simulink model "Tflex_PIDv1_ISSGP"  (R2018b)
settings: Solver=FixedStepDiscrete  StartTime=0.0  StopTime=inf  FixedStep=ts  RelTol=1e-3  EnableMultiTasking=on
PreLoadFcn:
  | Ts = 0.001;
InitFcn:
  | Ts = 0.001;
values from neighbouring files (symbols this model uses):
  a0 = omega_n^3    (= 31006276.6803)    [init_Tflex_PID_ISSGP.m]
  a1 = 3*omega_n^2    (= 296088.132033)    [init_Tflex_PID_ISSGP.m]
  a2 = 3*omega_n    (= 942.477796077)    [init_Tflex_PID_ISSGP.m]
  Avout = 10000    [init_Tflex_PID_ISSGP.m]
  b = ones(2*D,Q)*0.001    [init_Tflex_PID_ISSGP.m]
  D = 30    [init_Tflex_PID_ISSGP.m]
  FB1_offset = 1411500000    [init_Tflex_PID_ISSGP.m]
  h = 10*ts    (= 0.01)    [init_Tflex_PID_ISSGP.m]
  I_limit_max = 750    [init_Tflex_PID_ISSGP.m]
  I_limit_min = -250    [init_Tflex_PID_ISSGP.m]
  Kd = kp*(tau_z-tau_p*(1+(tau_z+tau_p)/tau_i))    [init_Tflex_PID_ISSGP.m]
  Ki = kp/tau_i    [init_Tflex_PID_ISSGP.m]
  Kp = kp*(1+(tau_z-tau_p)/tau_i)    [init_Tflex_PID_ISSGP.m]
  kp = m_eq*crossOver^2/sqrt(1/alpha)    [init_Tflex_PID_ISSGP.m]
  KTY_p0 = -146    [init_Tflex_PID_ISSGP.m]
  KTY_p1 = 263.3    [init_Tflex_PID_ISSGP.m]
  r = 1e2    (= 100)    [init_Tflex_PID_ISSGP.m]
  R = eye(2*D,2*D)*sn    [init_Tflex_PID_ISSGP.m]
  seed = 48125    [init_Tflex_PID_ISSGP.m]
  sf = 1.666976616732943e+05    (= 166697.661673)    [init_Tflex_PID_ISSGP.m]    (also in plot_Tflex_PIDv1_ISSGP18a.m = 500)
  sp_ts = 2    [init_Tflex_PID_ISSGP.m]
  tau_i = beta*tau_z    [init_Tflex_PID_ISSGP.m]
  tau_p = 1/(crossOver*sqrt(1/alpha))    [init_Tflex_PID_ISSGP.m]
  tau_z = sqrt(1/alpha)/crossOver    [init_Tflex_PID_ISSGP.m]
  tm = 1.5    [init_Tflex_PID_ISSGP.m]
  ts = 1/fs    (= 0.001)    [init_Tflex_PID_ISSGP.m]
  w = ones(2*D,Q)*0.001    [init_Tflex_PID_ISSGP.m]
undefined symbols (not defined in the file or in its folder): DiscIntNeverNeededParam, LPden, LPnum, SIGMA
libraries: xpcethercatlib x17, simulink x10, slrtlib x5
settings Model: SimulationMode=external  ExtModeTrigDirection=either  Creator=lab  LastModifiedBy=wout7
settings SolverCC: ConcurrentTasks=on  AutoInsertRateTranBlk=on
settings DataIOCC: LimitDataPoints=on  MaxDataPoints=50000  SaveFormat=StructureWithTime
settings OptimizationCC: BlockReduction=off  OptimizeBlockIOStorage=off  BufferReuse=off  GlobalBufferReuse=off  ExpressionFolding=off  LocalBlockOutputs=off  OptimizeDataStoreBuffers=off  BusAssignmentInplaceUpdate=off
settings DebuggingCC: UnconnectedInputMsg=none  UnconnectedOutputMsg=none  UnconnectedLineMsg=none  LibraryContextMissingDiagnostic=none
settings HardwareCC: ProdBitPerPointer=32  ProdBitPerSizeT=32  ProdBitPerPtrDiffT=32  ProdLargestAtomicFloat=None  ProdWordSize=32  ProdLongLongMode=on  ProdHWDeviceType=Generic->32-bit x86 compatible
settings SFSimCC: SimUserSources=dpotrs_wrapper.c;  SimUserLibraries=libmwlapack.lib  SimUseLocalCustomCode=off
settings SFSimCC: SimUserIncludeDirs=|
  | "C:\Program Files\MATLAB\R2018a\extern\lib\win64\microsoft"
  | "C:\Program Files\MATLAB\R2018a\bin\win64"
  | "C:\Users\wout7\Documents\GitHub\Inverse_dynamics_learning\TargetPC\Tflex PID 17-5-2019\TLC"
settings RTWCC: SystemTargetFile=slrt.tlc  TemplateMakefile=slrt_default_tmf  Description=Simulink Real-Time  RTWUseLocalCustomCode=off  CodeExecutionProfiling=on  RTWCompilerOptimization=on
settings SimulinkRealTimeCC: SupportVariableSizeSignals=on  PreserveStateflowLocalDataDimensions=off  xPCConcurrentTasks=on

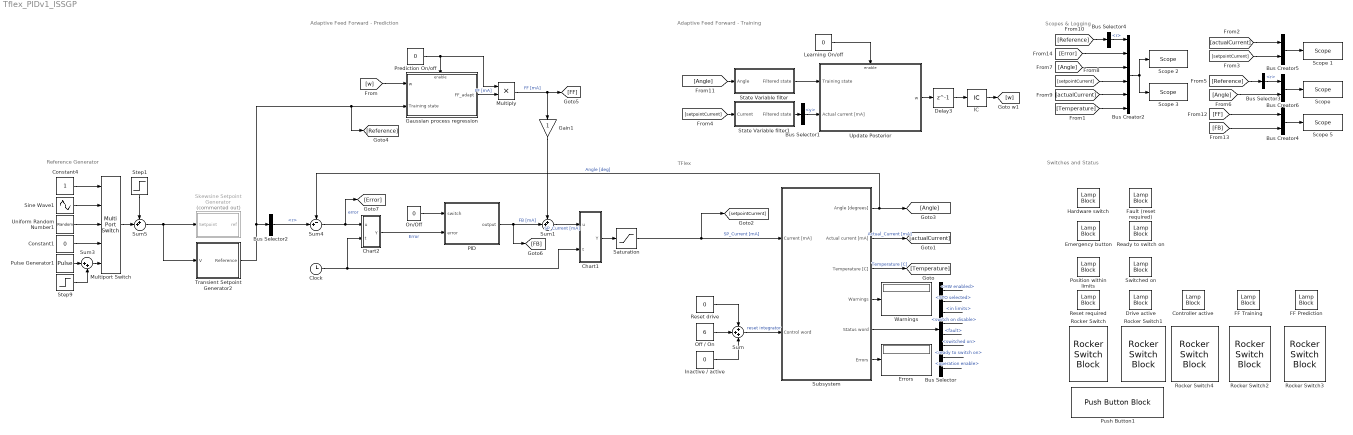
== system Tflex_PIDv1_ISSGP ==
  note: TFlex
  note: Switches and Status
  note: Scopes & Logging
  note: Adaptive Feed Forward - Prediction
  note: Reference Generator
  note: Adaptive Feed Forward - Training
  Bus Creator2 : BusCreator  Inputs=6
  Bus Creator4 : BusCreator  Inputs=2
  Bus Creator5 : BusCreator  Inputs=2
  Bus Creator6 : BusCreator  Inputs=2
  Bus Selector : BusSelector  OutputSignals=HW enabled,STO selected,in limits,switch on disable,fault,switched on,ready to switch on,operation enable
  Bus Selector1 : BusSelector  OutputSignals=y
  Bus Selector2 : BusSelector  OutputSignals=r
  Bus Selector3 : BusSelector  OutputSignals=r
  Bus Selector4 : BusSelector  OutputSignals=r
  Chart1 : Stateflow chart  TreatAsAtomicUnit=on
  Chart2 : Stateflow chart  TreatAsAtomicUnit=on
  Clock : Clock
  Constant1 : Constant  Value=0  SampleTime=sp_ts
  Constant4 : Constant  SampleTime=sp_ts
  Controller active : LampBlock  WebBlockId=1912  LabelPosition=Hide
  Delay3 : Delay  DelayLength=1  InitialCondition=0
  Drive active : LampBlock  WebBlockId=227
  Emergency button : LampBlock  WebBlockId=221
  Errors : Display
  FF Prediction : LampBlock  WebBlockId=1916  LabelPosition=Hide
  FF Training : LampBlock  WebBlockId=1915  LabelPosition=Hide
  Fault (reset required) : LampBlock  WebBlockId=224
  Gain1 : Gain
  Gaussian process regression : Subsystem
  Hardware switch : LampBlock  WebBlockId=218
  IC : InitialCondition  Value=w
  Inactive / active : Constant  Value=0
  Learning On/off : Constant  Value=0
  Multiply : Product
  Multiport Switch : MultiPortSwitch  Inputs=4
  Off / On : Constant  Value=6
  On/Off : Constant  Value=0
  "PID " : Subsystem
  Position within limits : LampBlock  WebBlockId=222
  Prediction On/off : Constant  Value=0  SampleTime=ts
  Pulse Generator1 : DiscretePulseGenerator  Amplitude=46  SampleTime=sp_ts
  Push Button1 : PushButtonBlock  WebBlockId=1977  ButtonText=Reset Drive [TURN OFF FIRST]  OnValue=128
  Ready to switch on : LampBlock  WebBlockId=226
  Reset drive : Constant  Value=0
  Reset required : LampBlock  WebBlockId=223
  Rocker Switch : RockerSwitchBlock  WebBlockId=231  LabelPosition=Hide
      settings: Values={{'Off', 'Driver On'}, [6 7]}
  Rocker Switch1 : RockerSwitchBlock  WebBlockId=232  LabelPosition=Hide
      settings: Values={{'Inactive', 'Driver Active'}, [0 8]}
  Rocker Switch2 : RockerSwitchBlock  WebBlockId=965  LabelPosition=Hide
      settings: Values={{'Off', 'Training on'}, [0 1]}
  Rocker Switch3 : RockerSwitchBlock  WebBlockId=969  LabelPosition=Hide
      settings: Values={{'Off', 'Prediction On'}, [0 1]}
  Rocker Switch4 : RockerSwitchBlock  WebBlockId=1848  LabelPosition=Hide
      settings: Values={{'Off', 'Controller On'}, [0 1]}
  Saturation : Saturate  UpperLimit=750  LowerLimit=-250/2
  "Scope " : slrtlib/Displays and Logging/Scope   scopeno=1  scopetype=Target  autostart=on  viewmode=Graphical redraw  formatstr='%15.6f'  grid=on  ylimits=[0 ,0]  nosamples=2000  noprepostsamples=0  interleave=1  triggermode=FreeRun  triggersignal=1  trigsignalfromport=off  triggerlevel=0.0  triggerslope=Either  triggerscope=1  triggersample=0  filename=data.dat  mode=Lazy  writesize=512  autorestart=off  dynamicfilemode=off  maxwritefilesize=512*1024^2
  Scope 1 : slrtlib/Displays and Logging/Scope   scopeno=2  scopetype=Target  autostart=on  viewmode=Graphical redraw  formatstr='%15.6f'  grid=on  ylimits=[500,500]  nosamples=250  noprepostsamples=0  interleave=1  triggermode=FreeRun  triggersignal=1  trigsignalfromport=off  triggerlevel=0.0  triggerslope=Either  triggerscope=1  triggersample=0  filename=data.dat  mode=Lazy  writesize=512  autorestart=off  dynamicfilemode=off  maxwritefilesize=512*1024^2
  Scope 2 : slrtlib/Displays and Logging/Scope   scopeno=3  scopetype=Target  autostart=on  viewmode=Numerical  formatstr='%15.6f,%15.6f,%15.6f,%15.0f'  grid=on  ylimits=[500,500]  nosamples=250  noprepostsamples=0  interleave=1  triggermode=FreeRun  triggersignal=1  trigsignalfromport=off  triggerlevel=0.0  triggerslope=Either  triggerscope=1  triggersample=0  filename=data.dat  mode=Lazy  writesize=512  autorestart=off  dynamicfilemode=off  maxwritefilesize=512*1024^2
  Scope 3 : slrtlib/Displays and Logging/Scope   scopeno=6  scopetype=File  autostart=on  viewmode=Graphical redraw  formatstr='%15.6f'  grid=on  ylimits=[0,0]  nosamples=600000  noprepostsamples=0  interleave=1  triggermode=FreeRun  triggersignal=1  trigsignalfromport=off  triggerlevel=0.0  triggerslope=Either  triggerscope=1  triggersample=0  filename=data.dat  mode=Lazy  writesize=512  autorestart=off  dynamicfilemode=off  maxwritefilesize=512*1024^2
  Scope 5 : slrtlib/Displays and Logging/Scope   scopeno=5  scopetype=Target  autostart=on  viewmode=Graphical redraw  formatstr='%15.6f'  grid=on  ylimits=[500,500]  nosamples=250  noprepostsamples=0  interleave=1  triggermode=FreeRun  triggersignal=1  trigsignalfromport=off  triggerlevel=0.0  triggerslope=Either  triggerscope=1  triggersample=0  filename=data.dat  mode=Lazy  writesize=512  autorestart=off  dynamicfilemode=off  maxwritefilesize=512*1024^2
  Sine Wave1 : Sin  Amplitude=15  Frequency=2*pi*2  SampleTime=0
  Skewsine Setpoint Generator : Subsystem  Commented=on
  State Variable filter : Subsystem
  State Variable filter1 : Subsystem
  Step1 : Step  Time=20  Before=-23  After=0  SampleTime=0
  Step9 : Step  Time=0  After=-24  SampleTime=sp_ts
  Subsystem : Subsystem
  Sum : Sum  Inputs=+++
  Sum1 : Sum  Inputs=++|
  Sum3 : Sum  Inputs=|++
  Sum4 : Sum  Inputs=-+|
  Sum5 : Sum  Inputs=++|
  Switched on : LampBlock  WebBlockId=225
  Transient Setpoint Generator2 : Subsystem
  Uniform Random Number1 : UniformRandomNumber  Seed=seed  SampleTime=sp_ts
  Update Posterior : Subsystem
  Warnings : Display
  wires:
  Subsystem/2(Actual current [mA]) -> [actualCurrent]  "Actual_Current [mA]"
  Subsystem/5(Status word) -> Bus Selector/1
  Bus Selector/1 -> ?  "<HW enabled>"
  Bus Selector/2 -> ?  "<STO selected>"
  Bus Selector/3 -> ?  "<in limits>"
  Bus Selector/4 -> ?  "<switch on disable>"
  Bus Selector/5 -> ?  "<fault>"
  Bus Selector/6 -> ?  "<switched on>"
  Bus Selector/7 -> ?  "<ready to switch on>"
  Bus Selector/8 -> ?  "<operation enable>"
  Reset drive/1 -> Sum/1
  Off / On/1 -> Sum/2
  Inactive / active/1 -> Sum/3
  Subsystem/3(Temperature [C]) -> [Temperature]  "Temperature [C]"
  Subsystem/4(Warnings) -> Warnings/1
  Subsystem/6(Errors) -> Errors/1
  Sum/1 -> Subsystem/2(Control word)  "reset integrator"
  Subsystem/1(Angle [degrees]) -> [Angle], Sum4/1  "Angle [deg]"
  Chart1/1(Y) -> Saturation/1
  Sum1/1 -> Chart1/1(u)  "SP_Current [mA]"
  Chart2/1(Y) -> "PID "/2(error)  "Error"
  Sum4/1 -> [Error], Chart2/1(u)  "error"
  Clock/1 -> Chart2/2(t), Chart1/2(t)
  State Variable filter/1(Filtered state) -> Update Posterior/1(Training state)
  IC/1 -> [w]
  Delay3/1 -> IC/1
  Update Posterior/1(w) -> Delay3/1
  [w] -> Gaussian process regression/1(w)
  Prediction On/off/1 -> Gaussian process regression/Enable, Multiply/1
  Learning On/off/1 -> Update Posterior/Enable
  Bus Creator4/1 -> Scope 5/1
  Uniform Random Number1/1 -> Multiport Switch/3
  Sine Wave1/1 -> Multiport Switch/2
  Constant4/1 -> Multiport Switch/1
  Transient Setpoint Generator2/1(Reference) -> Gaussian process regression/2(Training state), [Reference], Bus Selector2/1
  Sum5/1 -> Skewsine Setpoint Generator/1(Setpoint), Transient Setpoint Generator2/1(V)
  Gain1/1 -> Sum1/1
  Multiply/1 -> Gain1/1, [FF]  "FF [mA]"
  Gaussian process regression/1(FF_adapt) -> Multiply/2  "FF [mA]"
  State Variable filter1/1(Filtered state) -> Bus Selector1/1
  Bus Selector1/1 -> Update Posterior/2("Actual current [mA] ")  "<y>"
  [setpointCurrent] -> State Variable filter1/1(Current)
  [actualCurrent] -> Bus Creator5/1
  [setpointCurrent] -> Bus Creator5/2
  Bus Creator5/1 -> Scope 1/1
  [Reference] -> Bus Selector3/1
  [Angle] -> Bus Creator6/2
  Bus Selector3/1 -> Bus Creator6/1  "<r>"
  Bus Creator6/1 -> "Scope "/1
  [Reference] -> Bus Selector4/1
  [Angle] -> Bus Creator2/3
  [setpointCurrent] -> Bus Creator2/4
  [actualCurrent] -> Bus Creator2/5
  [Temperature] -> Bus Creator2/6
  Bus Creator2/1 -> Scope 2/1, Scope 3/1
  [Angle] -> State Variable filter/1(Angle)
  "PID "/1(output) -> [FB], Sum1/2  "FB [mA]"
  [FF] -> Bus Creator4/1
  [FB] -> Bus Creator4/2
  Bus Selector2/1 -> Sum4/2  "<r>"
  [Error] -> Bus Creator2/2
  Saturation/1 -> [setpointCurrent], Subsystem/1(Current [mA])  "SP_Current [mA]"
  Bus Selector4/1 -> Bus Creator2/1  "<r>"
  On/Off/1 -> "PID "/1(switch)
  Multiport Switch/1 -> Sum5/2
  Step1/1 -> Sum5/1
  Pulse Generator1/1 -> Sum3/1
  Step9/1 -> Sum3/2
  Sum3/1 -> Multiport Switch/5
  Constant1/1 -> Multiport Switch/4

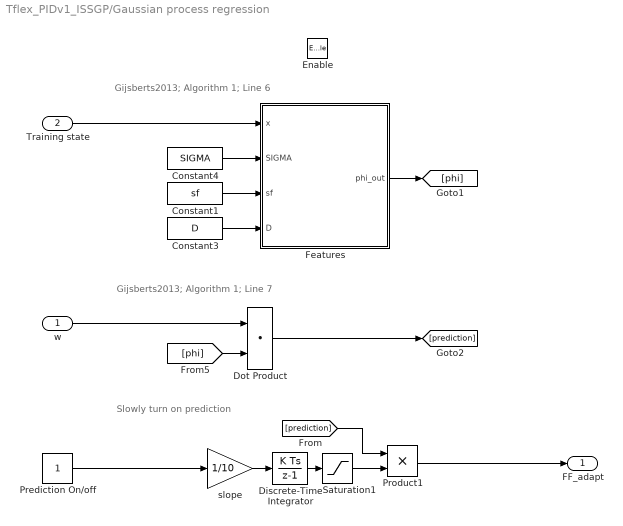
== system Tflex_PIDv1_ISSGP/Gaussian process regression ==
  note: Gijsberts2013; Algorithm 1; Line 7
  note: Gijsberts2013; Algorithm 1; Line 6
  note: Slowly turn on prediction
  w : Inport
  Training state : Inport  Port=2
  Enable : EnablePort  StatesWhenEnabling=reset
  Constant1 : Constant  Value=sf  VectorParams1D=off
  Constant3 : Constant  Value=D  VectorParams1D=off
  Constant4 : Constant  Value=SIGMA  VectorParams1D=off
  Discrete-Time Integrator : DiscreteIntegrator  SampleTime=-1  ICPrevOutput=DiscIntNeverNeededParam  ICPrevScaledInput=DiscIntNeverNeededParam
  Dot Product : DotProduct  OutDataTypeStr=Inherit: Inherit via internal rule
  Features : Subsystem
  Prediction On/off : Constant
  Product1 : Product
  Saturation1 : Saturate  UpperLimit=1  LowerLimit=0
  slope : Gain  Gain=1/10
  FF_adapt : Outport  SampleTime=ts
  wires:
  w/1 -> Dot Product/1
  [phi] -> Dot Product/2
  Product1/1 -> FF_adapt/1
  slope/1 -> Discrete-Time Integrator/1
  Prediction On/off/1 -> slope/1
  Discrete-Time Integrator/1 -> Saturation1/1
  Dot Product/1 -> [prediction]
  Constant4/1 -> Features/2(SIGMA)
  Training state/1 -> Features/1(x)
  Features/1(phi_out) -> [phi]
  Constant3/1 -> Features/4(D)
  Constant1/1 -> Features/3(sf)
  Saturation1/1 -> Product1/2
  [prediction] -> Product1/1

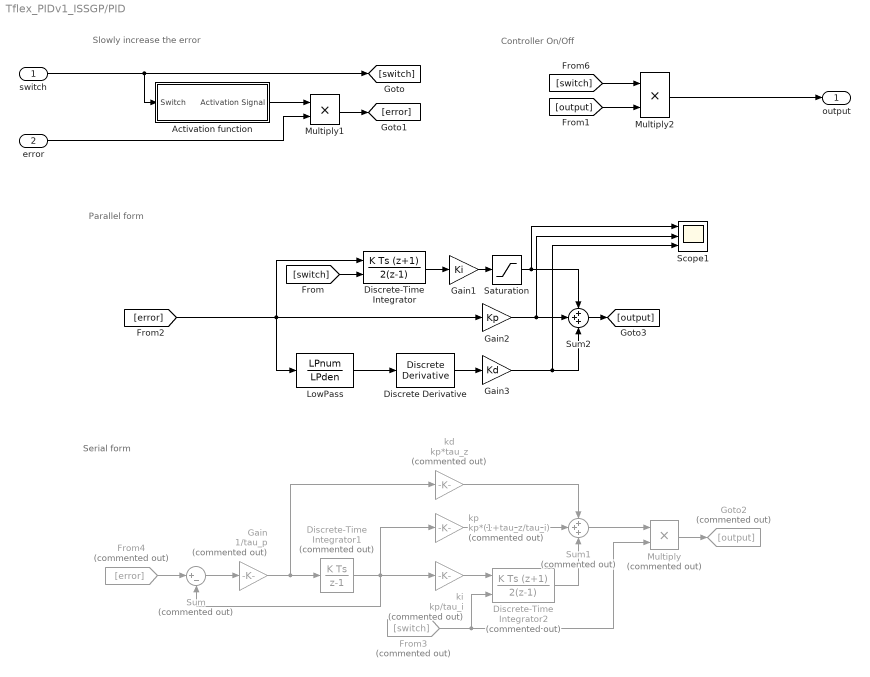
== system Tflex_PIDv1_ISSGP/PID  ==
  note: Controller On/Off
  note: Slowly increase the error
  note: Serial form
  note: Parallel form
  switch : Inport  SampleTime=ts
  error : Inport  Port=2
  Activation function : Subsystem
  Discrete Derivative : simulink/Discrete/Discrete Derivative  gainval=1.0  ICPrevScaledInput=0.0  OutMin=[]  OutMax=[]  OutDataType=fixdt(1, 16)  OutScaling=2^-10  DoSatur=off
  Discrete-Time Integrator : DiscreteIntegrator  IntegratorMethod=Integration: Trapezoidal  ExternalReset=either  SampleTime=ts  LimitOutput=on  UpperSaturationLimit=I_limit_max  LowerSaturationLimit=I_limit_min  ICPrevOutput=DiscIntNeverNeededParam  ICPrevScaledInput=DiscIntNeverNeededParam
  Discrete-Time Integrator1 : DiscreteIntegrator  Commented=on  SampleTime=-1  ICPrevOutput=DiscIntNeverNeededParam  ICPrevScaledInput=DiscIntNeverNeededParam
  Discrete-Time Integrator2 : DiscreteIntegrator  Commented=on  IntegratorMethod=Integration: Trapezoidal  ExternalReset=rising  SampleTime=ts  LimitOutput=on  UpperSaturationLimit=I_limit_max  LowerSaturationLimit=I_limit_min  ICPrevOutput=DiscIntNeverNeededParam  ICPrevScaledInput=DiscIntNeverNeededParam
  From3 : From  Commented=on  GotoTag=switch
  From4 : From  Commented=on  GotoTag=error
  Gain : Gain  Commented=on  Gain=1/tau_p
  Gain1 : Gain  Gain=Ki
  Gain2 : Gain  Gain=Kp
  Gain3 : Gain  Gain=Kd
  Goto2 : Goto  Commented=on  GotoTag=output
  LowPass : DiscreteTransferFcn  Numerator=LPnum  Denominator=LPden
  Multiply : Product  Commented=on
  Multiply1 : Product
  Multiply2 : Product
  Saturation : Saturate  UpperLimit=I_limit_max  LowerLimit=I_limit_min
  Scope1 : Scope  NumInputPorts=3
  Sum : Sum  Commented=on  Inputs=|+-
  Sum1 : Sum  Commented=on  Inputs=+++
  Sum2 : Sum  Inputs=+++
  kd : Gain  Commented=on  Gain=kp*tau_z
  ki : Gain  Commented=on  Gain=kp/tau_i
  kp : Gain  Commented=on  Gain=kp*(1+tau_z/tau_i)
  output : Outport
  wires:
  LowPass/1 -> Discrete Derivative/1
  [error] -> Discrete-Time Integrator/1, Gain2/1, LowPass/1
  Discrete-Time Integrator/1 -> Gain1/1
  Gain2/1 -> Scope1/2, Sum2/2
  Gain3/1 -> Scope1/3, Sum2/3
  Sum2/1 -> [output]
  Sum/1 -> Gain/1
  Gain/1 -> Discrete-Time Integrator1/1, kd/1
  ki/1 -> Discrete-Time Integrator2/1
  Discrete-Time Integrator1/1 -> kp/1, ki/1, Sum/2
  kp/1 -> Sum1/2
  kd/1 -> Sum1/1
  Discrete-Time Integrator2/1 -> Sum1/3
  Discrete Derivative/1 -> Gain3/1
  From4/1 -> Sum/1
  Sum1/1 -> Multiply/1
  From3/1 -> Discrete-Time Integrator2/2, Multiply/2
  Multiply/1 -> Goto2/1
  switch/1 -> [switch], Activation function/1(Switch)
  error/1 -> Multiply1/2
  [output] -> Multiply2/2
  [switch] -> Discrete-Time Integrator/2
  Multiply1/1 -> [error]
  [switch] -> Multiply2/1
  Multiply2/1 -> output/1
  Saturation/1 -> Sum2/1, Scope1/1
  Gain1/1 -> Saturation/1
  Activation function/1(Activation Signal) -> Multiply1/1

== system Tflex_PIDv1_ISSGP/Skewsine Setpoint Generator ==
  Setpoint : Inport
  Bus Creator : BusCreator  Inputs=3
  Delay : Delay  Commented=through  DelayLength=1  InitialCondition=0
  Subsystem : Subsystem
  ref : Outport
  wires:
  Subsystem/3(r_ddot) -> Bus Creator/3  "r_ddot"
  Bus Creator/1 -> ref/1
  Setpoint/1 -> Delay/1
  Subsystem/2(r_dot) -> Bus Creator/2  "r_dot"
  Subsystem/1(r) -> Bus Creator/1  "r"
  Delay/1 -> Subsystem/1(setpoint)

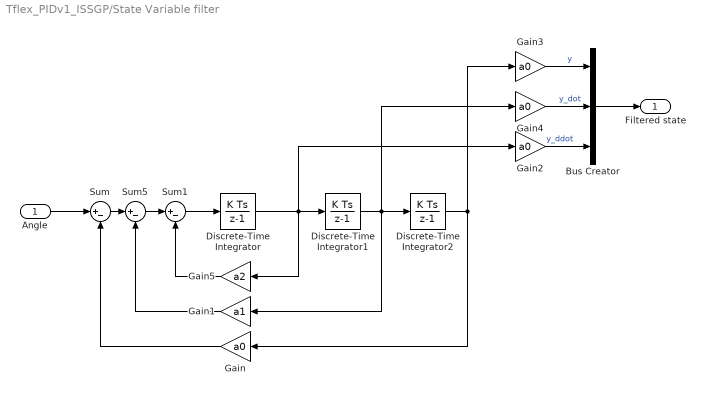
== system Tflex_PIDv1_ISSGP/State Variable filter ==
  Angle : Inport
  Bus Creator : BusCreator  Inputs=3
  Discrete-Time Integrator : DiscreteIntegrator  SampleTime=-1  ICPrevOutput=DiscIntNeverNeededParam  ICPrevScaledInput=DiscIntNeverNeededParam
  Discrete-Time Integrator1 : DiscreteIntegrator  SampleTime=-1  ICPrevOutput=DiscIntNeverNeededParam  ICPrevScaledInput=DiscIntNeverNeededParam
  Discrete-Time Integrator2 : DiscreteIntegrator  SampleTime=-1  ICPrevOutput=DiscIntNeverNeededParam  ICPrevScaledInput=DiscIntNeverNeededParam
  Gain{,2..4} (4 alike) : Gain  Gain=a0
  Gain1 : Gain  Gain=a1
  Gain5 : Gain  Gain=a2
  Sum : Sum  Inputs=|+-
  Sum1 : Sum  Inputs=|+-
  Sum5 : Sum  Inputs=|+-
  Filtered state : Outport
  wires:
  Bus Creator/1 -> Filtered state/1
  Angle/1 -> Sum/1
  Sum/1 -> Sum5/1
  Gain/1 -> Sum/2
  Gain1/1 -> Sum5/2
  Gain3/1 -> Bus Creator/1  "y"
  Gain2/1 -> Bus Creator/3  "y_ddot"
  Gain4/1 -> Bus Creator/2  "y_dot"
  Gain5/1 -> Sum1/2
  Sum5/1 -> Sum1/1
  Sum1/1 -> Discrete-Time Integrator/1
  Discrete-Time Integrator/1 -> Discrete-Time Integrator1/1, Gain2/1, Gain5/1
  Discrete-Time Integrator1/1 -> Discrete-Time Integrator2/1, Gain4/1, Gain1/1
  Discrete-Time Integrator2/1 -> Gain3/1, Gain/1

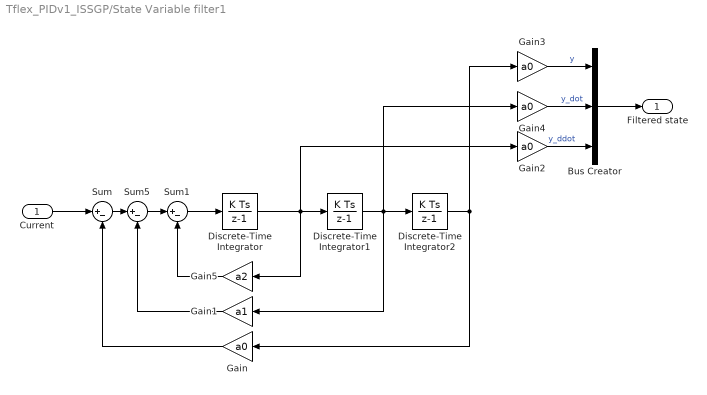
== system Tflex_PIDv1_ISSGP/State Variable filter1 ==
  Current : Inport
  Bus Creator : BusCreator  Inputs=3
  Discrete-Time Integrator : DiscreteIntegrator  SampleTime=-1  ICPrevOutput=DiscIntNeverNeededParam  ICPrevScaledInput=DiscIntNeverNeededParam
  Discrete-Time Integrator1 : DiscreteIntegrator  SampleTime=-1  ICPrevOutput=DiscIntNeverNeededParam  ICPrevScaledInput=DiscIntNeverNeededParam
  Discrete-Time Integrator2 : DiscreteIntegrator  SampleTime=-1  ICPrevOutput=DiscIntNeverNeededParam  ICPrevScaledInput=DiscIntNeverNeededParam
  Gain{,2..4} (4 alike) : Gain  Gain=a0
  Gain1 : Gain  Gain=a1
  Gain5 : Gain  Gain=a2
  Sum : Sum  Inputs=|+-
  Sum1 : Sum  Inputs=|+-
  Sum5 : Sum  Inputs=|+-
  Filtered state : Outport
  wires:
  Bus Creator/1 -> Filtered state/1
  Current/1 -> Sum/1
  Sum/1 -> Sum5/1
  Gain/1 -> Sum/2
  Gain1/1 -> Sum5/2
  Gain3/1 -> Bus Creator/1  "y"
  Gain2/1 -> Bus Creator/3  "y_ddot"
  Gain4/1 -> Bus Creator/2  "y_dot"
  Gain5/1 -> Sum1/2
  Sum5/1 -> Sum1/1
  Sum1/1 -> Discrete-Time Integrator/1
  Discrete-Time Integrator/1 -> Discrete-Time Integrator1/1, Gain2/1, Gain5/1
  Discrete-Time Integrator1/1 -> Discrete-Time Integrator2/1, Gain4/1, Gain1/1
  Discrete-Time Integrator2/1 -> Gain3/1, Gain/1

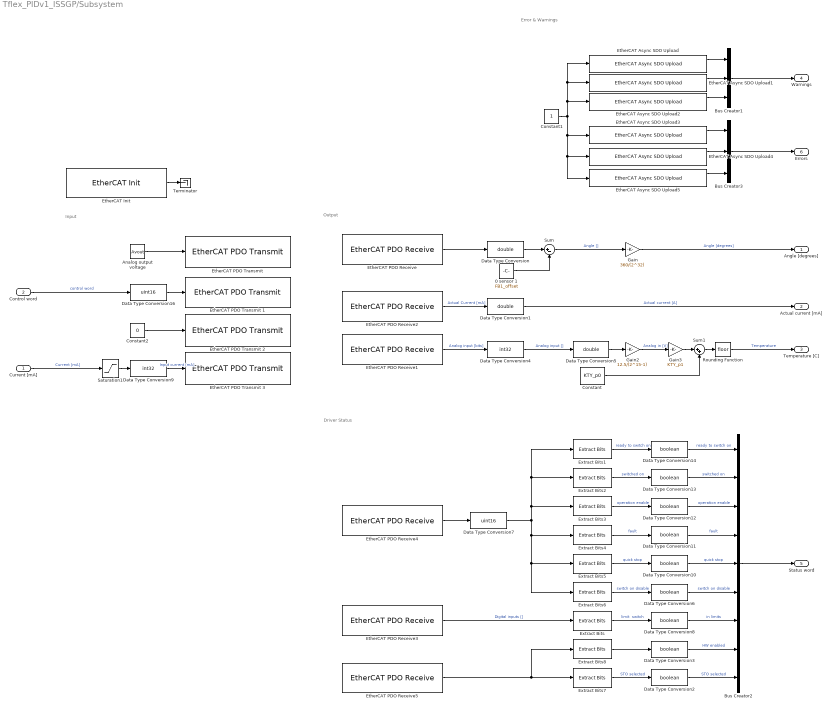
== system Tflex_PIDv1_ISSGP/Subsystem ==
  note: Output
  note: Error & Warnings
  note: Driver Status
  note: Input
  Current [mA] : Inport
  Control word : Inport  Port=2
  0 sensor 1 : Constant  Value=FB1_offset
  Analog output voltage : Constant  Value=Avout  OutDataTypeStr=int16
  Bus Creator1 : BusCreator  Inputs=3
  Bus Creator2 : BusCreator  Inputs=9
  Bus Creator3 : BusCreator  Inputs=3
  Constant : Constant  Value=KTY_p0
  Constant1 : Constant  OutDataTypeStr=int32
  Constant2 : Constant  Value=0  OutDataTypeStr=uint32
  Data Type Conversion : DataTypeConversion  OutDataTypeStr=double
  Data Type Conversion1 : DataTypeConversion  OutDataTypeStr=double
  Data Type Conversion{2..3,6,8,10..14} (9 alike) : DataTypeConversion  OutDataTypeStr=boolean
  Data Type Conversion16 : DataTypeConversion  OutDataTypeStr=uint16
  Data Type Conversion4 : DataTypeConversion  OutDataTypeStr=int32
  Data Type Conversion5 : DataTypeConversion  OutDataTypeStr=double
  Data Type Conversion7 : DataTypeConversion  OutDataTypeStr=uint16  RndMeth=Round
  Data Type Conversion9 : DataTypeConversion  OutDataTypeStr=int32
  EtherCAT Async SDO Upload : xpcethercatlib/EtherCAT Async SDO Upload  index=8192  subIndex=1  sig_type=uint32  sig_dim=1  device_id=0  slave_name=Drive 1 (AKD)  sample_time=1  slave_addr=1001  selected_slave=Term 1 (EK1100)  timeout=500  slave_found=1
      settings: SourceProductName=Simulink Real-Time  SourceProductBaseCode=XP
  EtherCAT Async SDO Upload1 : xpcethercatlib/EtherCAT Async SDO Upload  index=8192  subIndex=2  sig_type=uint32  sig_dim=1  device_id=0  slave_name=Drive 1 (AKD)  sample_time=1  slave_addr=1001  selected_slave=Term 1 (EK1100)  timeout=500  slave_found=1
      settings: SourceProductName=Simulink Real-Time  SourceProductBaseCode=XP
  EtherCAT Async SDO Upload2 : xpcethercatlib/EtherCAT Async SDO Upload  index=8192  subIndex=3  sig_type=uint32  sig_dim=1  device_id=0  slave_name=Drive 1 (AKD)  sample_time=1  slave_addr=1001  selected_slave=Term 1 (EK1100)  timeout=500  slave_found=1
      settings: SourceProductName=Simulink Real-Time  SourceProductBaseCode=XP
  EtherCAT Async SDO Upload3 : xpcethercatlib/EtherCAT Async SDO Upload  index=8193  subIndex=1  sig_type=uint32  sig_dim=1  device_id=0  slave_name=Drive 1 (AKD)  sample_time=1  slave_addr=1001  selected_slave=Term 1 (EK1100)  timeout=500  slave_found=1
      settings: SourceProductName=Simulink Real-Time  SourceProductBaseCode=XP
  EtherCAT Async SDO Upload4 : xpcethercatlib/EtherCAT Async SDO Upload  index=8193  subIndex=2  sig_type=uint32  sig_dim=1  device_id=0  slave_name=Drive 1 (AKD)  sample_time=1  slave_addr=1001  selected_slave=Term 1 (EK1100)  timeout=500  slave_found=1
      settings: SourceProductName=Simulink Real-Time  SourceProductBaseCode=XP
  EtherCAT Async SDO Upload5 : xpcethercatlib/EtherCAT Async SDO Upload  index=8193  subIndex=3  sig_type=uint32  sig_dim=1  device_id=0  slave_name=Drive 1 (AKD)  sample_time=1  slave_addr=1001  selected_slave=Term 1 (EK1100)  timeout=500  slave_found=1
      settings: SourceProductName=Simulink Real-Time  SourceProductBaseCode=XP
  "EtherCAT Init " : xpcethercatlib/EtherCAT Init   Priority=0  config_file=C:\Users\wout7\Documents\GitHub\Inverse_dynamics_learning\TargetPC\Tflex PID 17-5-2019\custom_pdo_eni3.xml  device_id=0  pci_bus=13  pci_slot=0  pci_function=0  initstate=2  dctuning=0  enaDebug=off  enaDC=on  errLink=off  masterDbg=off  stateChgDbg=off  baseClock=off  masterCfg=off  logFile='c:\dbglog.txt'  sample_time=0.001000  DCMode=2
      settings: SourceProductName=Simulink Real-Time  SourceProductBaseCode=XP
  EtherCAT PDO Receive : xpcethercatlib/EtherCAT PDO Receive  Priority=2  sig_name=Drive 1 (AKD).TPDO mapping parameter 3.Position actual internal value  sig_offset=624  sig_type=int32  type_size=32  sig_dim=1  device_id=0  sample_time=0.001000
      settings: SourceProductName=Simulink Real-Time  SourceProductBaseCode=XP
  EtherCAT PDO Receive1 : xpcethercatlib/EtherCAT PDO Receive  Priority=2  sig_name=Drive 1 (AKD).TPDO mapping parameter 1.AOUT_INPUT_VALUE  sig_offset=480  sig_type=int16  type_size=16  sig_dim=1  device_id=0  sample_time=0.001
      settings: SourceProductName=Simulink Real-Time  SourceProductBaseCode=XP
  EtherCAT PDO Receive2 : xpcethercatlib/EtherCAT PDO Receive  Priority=2  sig_name=Drive 1 (AKD).TPDO mapping parameter 2.Current actual value  sig_offset=528  sig_type=int32  type_size=32  sig_dim=1  device_id=0  sample_time=0.001000
      settings: SourceProductName=Simulink Real-Time  SourceProductBaseCode=XP
  EtherCAT PDO Receive3 : xpcethercatlib/EtherCAT PDO Receive  Priority=2  sig_name=Drive 1 (AKD).TPDO mapping parameter 1.Digital inputs  sig_offset=496  sig_type=uint32  type_size=32  sig_dim=1  device_id=0  sample_time=0.001000
      settings: SourceProductName=Simulink Real-Time  SourceProductBaseCode=XP
  EtherCAT PDO Receive4 : xpcethercatlib/EtherCAT PDO Receive  Priority=2  sig_name=Drive 1 (AKD).TPDO mapping parameter 1.Statusword  sig_offset=464  sig_type=uint16  type_size=16  sig_dim=1  device_id=0  sample_time=0.001
      settings: SourceProductName=Simulink Real-Time  SourceProductBaseCode=XP
  EtherCAT PDO Receive5 : xpcethercatlib/EtherCAT PDO Receive  Priority=2  sig_name=Drive 1 (AKD).TPDO mapping parameter 3.Manufacturer status register  sig_offset=592  sig_type=uint32  type_size=32  sig_dim=1  device_id=0  sample_time=0.001000
      settings: SourceProductName=Simulink Real-Time  SourceProductBaseCode=XP
  "EtherCAT PDO Transmit " : xpcethercatlib/EtherCAT PDO Transmit   Priority=3  sig_name=Drive 1 (AKD).RPDO mapping parameter 1.AOUT.VALUE write  sig_offset=480  sig_type=int16  type_size=16  sig_dim=1  device_id=0  sample_time=0.001000
      settings: SourceProductName=Simulink Real-Time  SourceProductBaseCode=XP
  EtherCAT PDO Transmit 1 : xpcethercatlib/EtherCAT PDO Transmit   Priority=3  sig_name=Drive 1 (AKD).RPDO mapping parameter 1.Controlword  sig_offset=464  sig_type=uint16  type_size=16  sig_dim=1  device_id=0  sample_time=0.001000
      settings: SourceProductName=Simulink Real-Time  SourceProductBaseCode=XP
  EtherCAT PDO Transmit 2 : xpcethercatlib/EtherCAT PDO Transmit   Priority=3  sig_name=Drive 1 (AKD).RPDO mapping parameter 1.Physical outputs  sig_offset=496  sig_type=uint32  type_size=32  sig_dim=1  device_id=0  sample_time=0.001000
      settings: SourceProductName=Simulink Real-Time  SourceProductBaseCode=XP
  EtherCAT PDO Transmit 3 : xpcethercatlib/EtherCAT PDO Transmit   Priority=3  sig_name=Drive 1 (AKD).RPDO mapping parameter 2.Target current  sig_offset=528  sig_type=int32  type_size=32  sig_dim=1  device_id=0  sample_time=0.001000
      settings: SourceProductName=Simulink Real-Time  SourceProductBaseCode=XP
  Extract Bits : simulink/Logic and Bit Operations/Extract Bits  bitsToExtract=Range of bits  numBits=8  bitIdxRange=[16]  outScalingMode=Treat bit field as an integer
      settings: SourceProductName=Simulink
  Extract Bits1 : simulink/Logic and Bit Operations/Extract Bits  bitsToExtract=Range of bits  numBits=8  bitIdxRange=[0]  outScalingMode=Treat bit field as an integer
      settings: SourceProductName=Simulink
  Extract Bits2 : simulink/Logic and Bit Operations/Extract Bits  bitsToExtract=Range of bits  numBits=8  bitIdxRange=[1]  outScalingMode=Treat bit field as an integer
      settings: SourceProductName=Simulink
  Extract Bits3 : simulink/Logic and Bit Operations/Extract Bits  bitsToExtract=Range of bits  numBits=8  bitIdxRange=[2]  outScalingMode=Treat bit field as an integer
      settings: SourceProductName=Simulink
  Extract Bits4 : simulink/Logic and Bit Operations/Extract Bits  bitsToExtract=Range of bits  numBits=8  bitIdxRange=[3]  outScalingMode=Treat bit field as an integer
      settings: SourceProductName=Simulink
  Extract Bits5 : simulink/Logic and Bit Operations/Extract Bits  bitsToExtract=Range of bits  numBits=8  bitIdxRange=[5]  outScalingMode=Treat bit field as an integer
      settings: SourceProductName=Simulink
  Extract Bits6 : simulink/Logic and Bit Operations/Extract Bits  bitsToExtract=Range of bits  numBits=8  bitIdxRange=[6]  outScalingMode=Treat bit field as an integer
      settings: SourceProductName=Simulink
  Extract Bits7 : simulink/Logic and Bit Operations/Extract Bits  bitsToExtract=Range of bits  numBits=8  bitIdxRange=[13]  outScalingMode=Treat bit field as an integer
      settings: SourceProductName=Simulink
  Extract Bits8 : simulink/Logic and Bit Operations/Extract Bits  bitsToExtract=Range of bits  numBits=8  bitIdxRange=[29]  outScalingMode=Treat bit field as an integer
      settings: SourceProductName=Simulink
  Gain : Gain  Gain=360/(2^32)
  Gain2 : Gain  Gain=12.5/(2^15-1)
  Gain3 : Gain  Gain=KTY_p1
  Rounding Function : Rounding
  Saturation1 : Saturate  UpperLimit=I_limit_max  LowerLimit=I_limit_min
  Sum : Sum  Inputs=|+-
  Sum1 : Sum  Inputs=|++  OutDataTypeStr=double
  Terminator : Terminator
  Angle [degrees] : Outport
  Actual current [mA] : Outport  Port=2
  Temperature [C] : Outport  Port=3
  Warnings : Outport  Port=4
  Status word : Outport  Port=5
  Errors : Outport  Port=6
  wires:
  Data Type Conversion/1 -> Sum/1
  Data Type Conversion9/1 -> EtherCAT PDO Transmit 3/1  "Input current [mA]"
  Bus Creator2/1 -> Status word/1
  0 sensor 1/1 -> Sum/2
  Data Type Conversion1/1 -> Actual current [mA]/1  "Actual current [A]"
  Data Type Conversion7/1 -> Extract Bits4/1, Extract Bits5/1, Extract Bits6/1, Extract Bits1/1, Extract Bits2/1, Extract Bits3/1
  EtherCAT PDO Receive4/1 -> Data Type Conversion7/1
  EtherCAT PDO Receive2/1 -> Data Type Conversion1/1  "Actual Current [mA]"
  Data Type Conversion4/1 -> Data Type Conversion5/1  "Analog input []"
  EtherCAT PDO Receive/1 -> Data Type Conversion/1
  Gain/1 -> Angle [degrees]/1  "Angle [degrees]"
  EtherCAT PDO Receive5/1 -> Extract Bits8/1, Extract Bits7/1
  EtherCAT PDO Receive1/1 -> Data Type Conversion4/1  "Analog input [bits]"
  Sum/1 -> Gain/1  "Angle []"
  Extract Bits8/1 -> Data Type Conversion3/1
  Extract Bits6/1 -> Data Type Conversion6/1  "switch on disable"
  Extract Bits/1 -> Data Type Conversion8/1  "limit  switch"
  Extract Bits3/1 -> Data Type Conversion12/1  "operation enable"
  Extract Bits2/1 -> Data Type Conversion13/1  "switched on"
  Extract Bits4/1 -> Data Type Conversion11/1  "fault"
  Extract Bits5/1 -> Data Type Conversion10/1  "quick stop"
  Constant2/1 -> EtherCAT PDO Transmit 2/1
  Extract Bits1/1 -> Data Type Conversion14/1  "ready to switch on"
  EtherCAT PDO Receive3/1 -> Extract Bits/1  "Digital inputs []"
  Extract Bits7/1 -> Data Type Conversion2/1  "STO selected"
  Data Type Conversion16/1 -> EtherCAT PDO Transmit 1/1
  "EtherCAT Init "/1 -> Terminator/1
  Data Type Conversion5/1 -> Gain2/1
  Analog output voltage/1 -> "EtherCAT PDO Transmit "/1
  Gain2/1 -> Gain3/1  "Analog in [V]"
  Sum1/1 -> Rounding Function/1
  Rounding Function/1 -> Temperature [C]/1  "Temperature"
  EtherCAT Async SDO Upload/1 -> Bus Creator1/1
  Bus Creator1/1 -> Warnings/1
  Constant1/1 -> EtherCAT Async SDO Upload5/1, EtherCAT Async SDO Upload4/1, EtherCAT Async SDO Upload3/1, EtherCAT Async SDO Upload/1, EtherCAT Async SDO Upload1/1, EtherCAT Async SDO Upload2/1
  EtherCAT Async SDO Upload1/1 -> Bus Creator1/2
  EtherCAT Async SDO Upload2/1 -> Bus Creator1/3
  EtherCAT Async SDO Upload3/1 -> Bus Creator3/1
  EtherCAT Async SDO Upload4/1 -> Bus Creator3/2
  EtherCAT Async SDO Upload5/1 -> Bus Creator3/3
  Bus Creator3/1 -> Errors/1
  Saturation1/1 -> Data Type Conversion9/1
  Gain3/1 -> Sum1/1
  Constant/1 -> Sum1/2
  Data Type Conversion8/1 -> Bus Creator2/7  "in limits"
  Data Type Conversion3/1 -> Bus Creator2/8  "HW enabled"
  Data Type Conversion10/1 -> Bus Creator2/5  "quick stop"
  Data Type Conversion6/1 -> Bus Creator2/6  "switch on disable"
  Data Type Conversion11/1 -> Bus Creator2/4  "fault"
  Data Type Conversion12/1 -> Bus Creator2/3  "operation enable"
  Data Type Conversion13/1 -> Bus Creator2/2  "switched on"
  Data Type Conversion2/1 -> Bus Creator2/9  "STO selected"
  Data Type Conversion14/1 -> Bus Creator2/1  "ready to switch on"
  Control word/1 -> Data Type Conversion16/1  "control word"
  Current [mA]/1 -> Saturation1/1  "Current [mA]"

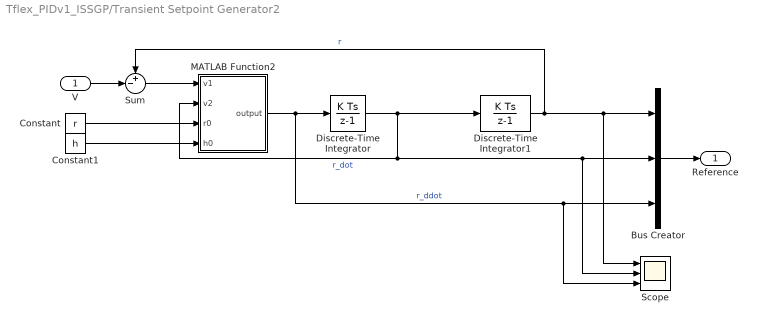
== system Tflex_PIDv1_ISSGP/Transient Setpoint Generator2 ==
  V : Inport
  Bus Creator : BusCreator  Inputs=3
  Constant : Constant  Value=r  SampleTime=ts
  Constant1 : Constant  Value=h  SampleTime=ts
  Discrete-Time Integrator : DiscreteIntegrator  gainval=1  SampleTime=ts  ICPrevOutput=DiscIntNeverNeededParam  ICPrevScaledInput=DiscIntNeverNeededParam
  Discrete-Time Integrator1 : DiscreteIntegrator  gainval=1  SampleTime=ts  ICPrevOutput=DiscIntNeverNeededParam  ICPrevScaledInput=DiscIntNeverNeededParam
  MATLAB Function2 : MATLAB Function  TreatAsAtomicUnit=on
  Scope : Scope  NumInputPorts=3
  Sum : Sum  Inputs=+-|
  Reference : Outport
  wires:
  Sum/1 -> MATLAB Function2/1(v1)
  V/1 -> Sum/2
  Constant/1 -> MATLAB Function2/3(r0)
  Constant1/1 -> MATLAB Function2/4(h0)
  Discrete-Time Integrator1/1 -> Scope/1, Bus Creator/1, Sum/1  "r"
  Discrete-Time Integrator/1 -> Discrete-Time Integrator1/1, MATLAB Function2/2(v2), Scope/2, Bus Creator/2  "r_dot"
  Bus Creator/1 -> Reference/1
  MATLAB Function2/1(output) -> Scope/3, Bus Creator/3, Discrete-Time Integrator/1  "r_ddot"

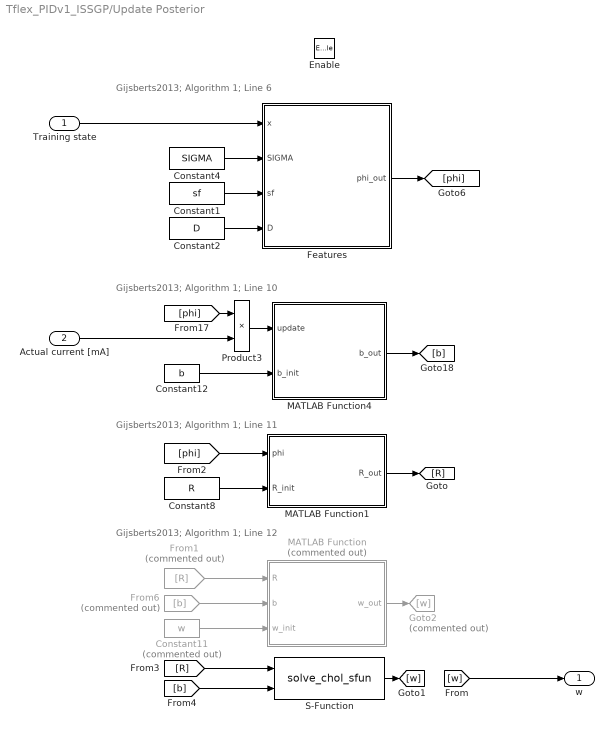
== system Tflex_PIDv1_ISSGP/Update Posterior ==
  note: Gijsberts2013; Algorithm 1; Line 6
  note: Gijsberts2013; Algorithm 1; Line 10
  note: Gijsberts2013; Algorithm 1; Line 11
  note: Gijsberts2013; Algorithm 1; Line 12
  Training state : Inport
  "Actual current [mA] " : Inport  Port=2
  Enable : EnablePort
  Constant1 : Constant  Value=sf  VectorParams1D=off
  Constant11 : Constant  Commented=on  Value=w  VectorParams1D=off  SampleTime=ts
  Constant12 : Constant  Value=b  VectorParams1D=off  SampleTime=ts
  Constant2 : Constant  Value=D  VectorParams1D=off
  Constant4 : Constant  Value=SIGMA  VectorParams1D=off
  Constant8 : Constant  Value=R  VectorParams1D=off  SampleTime=ts
  Features : Subsystem
  From1 : From  Commented=on  GotoTag=R
  From6 : From  Commented=on  GotoTag=b
  Goto2 : Goto  Commented=on  GotoTag=w
  MATLAB Function : MATLAB Function  Commented=on  TreatAsAtomicUnit=on
  MATLAB Function1 : MATLAB Function  TreatAsAtomicUnit=on
  MATLAB Function4 : MATLAB Function  TreatAsAtomicUnit=on
  Product3 : Product
  S-Function : S-Function  FunctionName=solve_chol_sfun  Parameters=2*D  SFunctionDeploymentMode=off  EnableBusSupport=off
  w : Outport
  wires:
  [phi] -> MATLAB Function1/1(phi)
  Training state/1 -> Features/1(x)
  Features/1(phi_out) -> [phi]
  MATLAB Function1/1(R_out) -> [R]
  Constant4/1 -> Features/2(SIGMA)
  From1/1 -> MATLAB Function/1(R)
  From6/1 -> MATLAB Function/2(b)
  Constant8/1 -> MATLAB Function1/2(R_init)
  Constant11/1 -> MATLAB Function/3(w_init)
  "Actual current [mA] "/1 -> Product3/2
  [phi] -> Product3/1
  Product3/1 -> MATLAB Function4/1(update)
  Constant12/1 -> MATLAB Function4/2(b_init)
  MATLAB Function4/1(b_out) -> [b]
  S-Function/1 -> [w]
  [w] -> w/1
  [R] -> S-Function/1
  [b] -> S-Function/2
  MATLAB Function/1(w_out) -> Goto2/1
  Constant1/1 -> Features/3(sf)
  Constant2/1 -> Features/4(D)

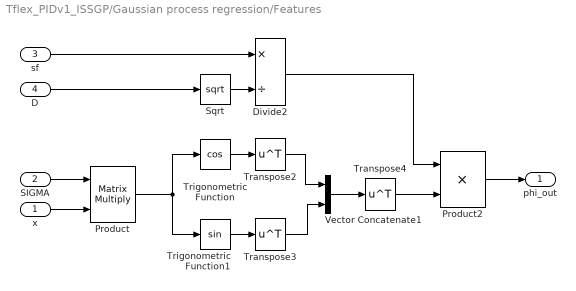
== system Tflex_PIDv1_ISSGP/Gaussian process regression/Features ==
  x : Inport
  SIGMA : Inport  Port=2
  sf : Inport  Port=3
  D : Inport  Port=4
  Divide2 : Product  Inputs=*/
  Product : Product  Multiplication=Matrix(*)
  Product2 : Product
  Sqrt : Sqrt  SaturateOnIntegerOverflow=on
  Transpose2 : Math  Operator=transpose  SaturateOnIntegerOverflow=on
  Transpose3 : Math  Operator=transpose  SaturateOnIntegerOverflow=on
  Transpose4 : Math  Operator=transpose  SaturateOnIntegerOverflow=on
  Trigonometric Function : Trigonometry  Operator=cos
  Trigonometric Function1 : Trigonometry
  Vector Concatenate1 : Concatenate
  phi_out : Outport
  wires:
  SIGMA/1 -> Product/1
  Product2/1 -> phi_out/1
  D/1 -> Sqrt/1
  Trigonometric Function1/1 -> Transpose3/1
  Trigonometric Function/1 -> Transpose2/1
  sf/1 -> Divide2/1
  Vector Concatenate1/1 -> Transpose4/1
  Transpose3/1 -> Vector Concatenate1/2
  Product/1 -> Trigonometric Function1/1, Trigonometric Function/1
  Divide2/1 -> Product2/1
  Transpose4/1 -> Product2/2
  Sqrt/1 -> Divide2/2
  Transpose2/1 -> Vector Concatenate1/1
  x/1 -> Product/2

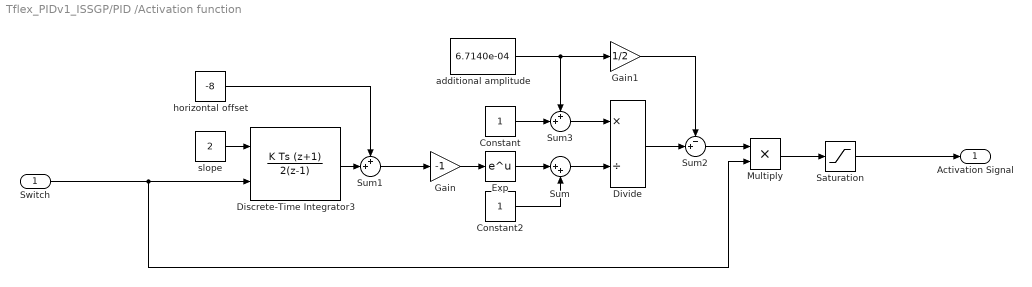
== system Tflex_PIDv1_ISSGP/PID /Activation function ==
  Switch : Inport
  Constant : Constant
  Constant2 : Constant
  Discrete-Time Integrator3 : DiscreteIntegrator  IntegratorMethod=Integration: Trapezoidal  ExternalReset=rising  SampleTime=-1  UpperSaturationLimit=1  LowerSaturationLimit=0  ICPrevOutput=DiscIntNeverNeededParam  ICPrevScaledInput=DiscIntNeverNeededParam
  Divide : Product  Inputs=*/
  Exp : Math  SaturateOnIntegerOverflow=on
  Gain : Gain  Gain=-1
  Gain1 : Gain  Gain=1/2
  Multiply : Product
  Saturation : Saturate  UpperLimit=1  LowerLimit=0
  Sum : Sum  Inputs=|++
  Sum1 : Sum  Inputs=++|
  Sum2 : Sum  Inputs=-+|
  Sum3 : Sum  Inputs=++|
  additional amplitude : Constant  Value=6.7140e-04
  horizontal offset : Constant  Value=-8
  slope : Constant  Value=2
  Activation Signal : Outport
  wires:
  Constant/1 -> Sum3/2
  Exp/1 -> Sum/1
  additional amplitude/1 -> Sum3/1, Gain1/1
  Sum1/1 -> Gain/1
  Gain1/1 -> Sum2/1
  Divide/1 -> Sum2/2
  Sum/1 -> Divide/2
  Gain/1 -> Exp/1
  slope/1 -> Discrete-Time Integrator3/1
  Discrete-Time Integrator3/1 -> Sum1/2
  Constant2/1 -> Sum/2
  Sum2/1 -> Multiply/1
  Sum3/1 -> Divide/1
  horizontal offset/1 -> Sum1/1
  Saturation/1 -> Activation Signal/1
  Multiply/1 -> Saturation/1
  Switch/1 -> Multiply/2, Discrete-Time Integrator3/2

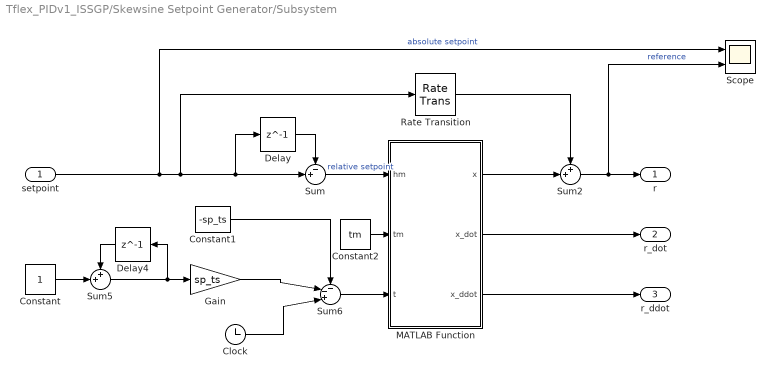
== system Tflex_PIDv1_ISSGP/Skewsine Setpoint Generator/Subsystem ==
  setpoint : Inport
  Clock : Clock
      settings: Decimation=100
  Constant : Constant  SampleTime=sp_ts
  Constant1 : Constant  Value=-sp_ts  SampleTime=sp_ts
  Constant2 : Constant  Value=tm  SampleTime=sp_ts
  Delay : Delay  DelayLength=1  InitialCondition=0  SampleTime=sp_ts
  Delay4 : Delay  DelayLength=1  InitialCondition=0  SampleTime=sp_ts
  Gain : Gain  Gain=sp_ts
  MATLAB Function : MATLAB Function  TreatAsAtomicUnit=on
  Rate Transition : RateTransition  OutPortSampleTime=ts
  Scope : Scope  NumInputPorts=2
  Sum : Sum  Inputs=-+|
  Sum2 : Sum  Inputs=++|
  Sum5 : Sum  Inputs=++|
  Sum6 : Sum  Inputs=--+|
  r : Outport
  r_dot : Outport  Port=2
  r_ddot : Outport  Port=3
  wires:
  Delay4/1 -> Sum5/1
  Sum2/1 -> r/1, Scope/2  "reference"
  Sum5/1 -> Delay4/1, Gain/1
  Constant/1 -> Sum5/2
  MATLAB Function/3(x_ddot) -> r_ddot/1
  Clock/1 -> Sum6/3
  Delay/1 -> Sum/1
  Gain/1 -> Sum6/2
  Constant1/1 -> Sum6/1
  MATLAB Function/2(x_dot) -> r_dot/1
  Sum/1 -> MATLAB Function/1(hm)  "relative setpoint"
  Constant2/1 -> MATLAB Function/2(tm)
  Sum6/1 -> MATLAB Function/3(t)
  MATLAB Function/1(x) -> Sum2/2
  setpoint/1 -> Scope/1, Rate Transition/1, Delay/1, Sum/2  "absolute setpoint"
  Rate Transition/1 -> Sum2/1

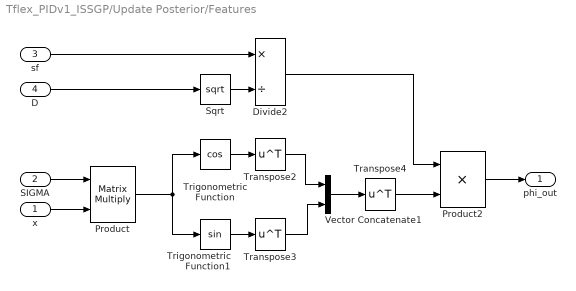
== system Tflex_PIDv1_ISSGP/Update Posterior/Features ==
  x : Inport
  SIGMA : Inport  Port=2
  sf : Inport  Port=3
  D : Inport  Port=4
  Divide2 : Product  Inputs=*/
  Product : Product  Multiplication=Matrix(*)
  Product2 : Product
  Sqrt : Sqrt  SaturateOnIntegerOverflow=on
  Transpose2 : Math  Operator=transpose  SaturateOnIntegerOverflow=on
  Transpose3 : Math  Operator=transpose  SaturateOnIntegerOverflow=on
  Transpose4 : Math  Operator=transpose  SaturateOnIntegerOverflow=on
  Trigonometric Function : Trigonometry  Operator=cos
  Trigonometric Function1 : Trigonometry
  Vector Concatenate1 : Concatenate
  phi_out : Outport
  wires:
  SIGMA/1 -> Product/1
  Product2/1 -> phi_out/1
  D/1 -> Sqrt/1
  Trigonometric Function1/1 -> Transpose3/1
  Trigonometric Function/1 -> Transpose2/1
  sf/1 -> Divide2/1
  Vector Concatenate1/1 -> Transpose4/1
  Transpose3/1 -> Vector Concatenate1/2
  Product/1 -> Trigonometric Function1/1, Trigonometric Function/1
  Divide2/1 -> Product2/1
  Transpose4/1 -> Product2/2
  Sqrt/1 -> Divide2/2
  Transpose2/1 -> Vector Concatenate1/1
  x/1 -> Product/2

== stateflow chart Tflex_PIDv1_ISSGP/Chart2 ==
  state ON
    Y=0;
  state OFF
    Y=0;
  state OFF1
    Y=u;
  (default) -> ON
  ON -> OFF : [u<90]
  OFF -> OFF1 [order 2] : [t>10]
  OFF -> ON [order 1] : [u>90]
  OFF1 -> OFF : [u>90]
  data: u input; Y output; t input

== matlab function Tflex_PIDv1_ISSGP/Update Posterior/MATLAB Function ==
  settings: updateMethod=DISCRETE  sampleTime=ts
  data: R input; w_out output; b input; w_init input
function w_out = updateW(R,b,w_init)
persistent w
if(isempty(w))
    w = w_init;
end
%coder.extrinsic('solve_chol');
%w = solve_chol(R,b);
w = R\(R'\b);
w_out = w;

== matlab function Tflex_PIDv1_ISSGP/Skewsine Setpoint Generator/Subsystem/MATLAB Function ==
  settings: updateMethod=DISCRETE  sampleTime=ts
  data: hm input; x output; tm input; t input; x_dot output; x_ddot output
function [x,x_dot,x_ddot] = skewSine(hm,tm,t)

if (t>=0) && (t<=tm)
    x      = hm/tm*t - hm/(2*pi)*sin(2*pi/tm*t);
    x_dot  = hm/tm - hm/tm*cos(2*pi/tm*t);
    x_ddot = 2*pi*hm/(tm^2)*sin(2*pi/tm*t);
else
    x      = hm;
    x_dot  = 0;
    x_ddot = 0;
end

== stateflow chart Tflex_PIDv1_ISSGP/Chart1 ==
  state OFF2
    Y=0;
  state ON
    Y=u;
  (default) -> OFF2
  OFF2 -> ON : [t>10]
  ON -> OFF2 : [t<10]
  data: u input; Y output; t input

== matlab function Tflex_PIDv1_ISSGP/Update Posterior/MATLAB Function1 ==
  settings: updateMethod=DISCRETE  sampleTime=ts
  data: R_out output; phi input; R_init input
function R_out = cholupdate_fcn(phi,R_init)
persistent R; 
if(isempty(R))
    R = R_init;
end
R = cholupdate(R,phi);
R_out = R;

== matlab function Tflex_PIDv1_ISSGP/Transient Setpoint Generator2/MATLAB Function2 ==
  data: v1 input; output output; v2 input; r0 input; h0 input
function output = Fhan(v1,v2,r0, h0)
d = h0^2*r0;
a0 = h0*v2;
y = v1 + a0;
a1 = sqrt(d*(d+8*abs(y)));
a2 = a0 + sign(y)*(a1-d)/2;
sy = (sign(y+d)-sign(y-d))/2;
a = (a0+y-a2)*sy +a2;
sa = (sign(a+d)-sign(a-d))/2;
output = -r0 *(a/d -sign(a) )*sa - r0*sign(a);

== matlab function Tflex_PIDv1_ISSGP/Update Posterior/MATLAB Function4 ==
  settings: updateMethod=DISCRETE  sampleTime=ts
  data: update input; b_out output; b_init input
function b_out = updateB(update, b_init)
persistent b 
if(isempty(b))
    b = b_init;
end

b = b + update;
b_out = b;
